simulink model "Main_model"  (R2021b)
settings: Solver=ode23t  StartTime=0.0  StopTime=sim_t_end  RelTol=1e-3
undefined symbols (not defined in the file): ambient_co2, ambient_pressure, ambient_rh, ambient_temp, battery, battery_heat_gen_scale, battery_mass, battery_thermal_mass, cab_air_v_dot, cabin_heater_cmd, cabin_heater_max_power, case_cold_plate_mass, case_cold_plate_thermal_mass, chiller_baffles_n, chiller_tube_length, chiller_tubes_n_rows, compressor_max_m_dot, compressor_ref_m_dot, condenser_air_min_flow_area, condenser_tube_width, const_current, coolant_channel_length, coolant_initial_T, coolant_m_dot, coolant_pipe_cross_sec_area, evaporator_air_cross_sec_area, evaporator_air_min_flow_area, evaporator_tube_width, motor_mc_heat_fraction, n_parallel, power_fraction_rear, ptc_heater_max_power, ptc_heater_thermal_mass, rad_air_v_dot, radiator_air_cross_sec_area, radiator_air_min_flow_area, radiator_tube_width, ref_m_dot, ref_pipe_dia, refrigerant_initial_void_fraction, refrigerant_pipe_cross_sec_area, T_bat_active_cool, T_bat_active_heat, T_bat_passive_cool, T_bat_passive_heat, T_battery_init, T_battery_nom, T_cabin_init, T_cabin_setpoint, T_dcdc_nom, T_DT_high, T_DT_passive_cool, T_DT_whr_active, T_front_gb_nom, T_front_mc_nom, T_front_motor_nom, T_rear_gb_nom, T_rear_mc_nom, T_rear_motor_nom, three_w_valve_max_open_area_factor ... (+3)
libraries: fl_lib x448, nesl_utility x328, SimscapeFluids_lib x134, slpidlib x15, ee_lib x9, simulink x8, LiBatteryElements_lib x4, SignalEditorBlockLib x1
(part 21 of 24)

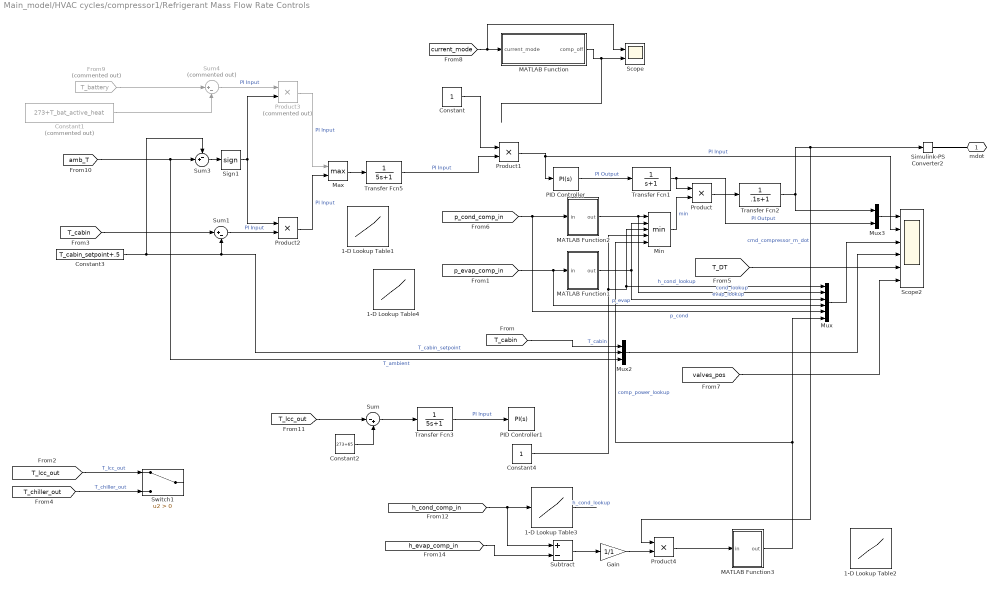
== system Main_model/HVAC cycles/compressor1/Refrigerant Mass Flow Rate Controls  ==
  1-D Lookup Table1 : Lookup_n-D  NumberOfTableDimensions=1  BreakpointsForDimension1=[0,2,2.75,5]  Table=[1,1,0,0]  InternalRulePriority=Speed  RndMeth=Simplest  InputSameDT=on
  1-D Lookup Table2 : Lookup_n-D  NumberOfTableDimensions=1  BreakpointsForDimension1=[0,7.5,8.5,10]  Table=[1,1,0,0]  InternalRulePriority=Speed  RndMeth=Simplest  InputSameDT=on
  1-D Lookup Table3 : Lookup_n-D  NumberOfTableDimensions=1  BreakpointsForDimension1=[400,445,465,500]  Table=[1,1,0,0]  InternalRulePriority=Speed  RndMeth=Simplest  InputSameDT=on
  1-D Lookup Table4 : Lookup_n-D  NumberOfTableDimensions=1  BreakpointsForDimension1=[0,0.08,0.15,1]  Table=[0,0,1,1]  InternalRulePriority=Speed  RndMeth=Simplest  InputSameDT=on
  Constant : Constant
  Constant1 : Constant  Commented=on  Value=273+T_bat_active_heat
  Constant2 : Constant  Value=273+65
  Constant3 : Constant  Value=T_cabin_setpoint+.5
  Constant4 : Constant
  From9 : From  Commented=on  GotoTag=T_battery
  Gain : Gain  Gain=1/1
  MATLAB Function : MATLAB Function  TreatAsAtomicUnit=on
  MATLAB Function1 : MATLAB Function  TreatAsAtomicUnit=on
  MATLAB Function2 : MATLAB Function  TreatAsAtomicUnit=on
  MATLAB Function3 : MATLAB Function  TreatAsAtomicUnit=on
  Max : MinMax  Function=max  Inputs=2
  Min : MinMax  Inputs=5
  Mux : Mux  Inputs=6
  Mux2 : Mux  Inputs=3
  Mux3 : Mux  Inputs=2
  PID Controller : slpidlib/PID Controller  Controller=PI  Form=Parallel  TimeDomain=Continuous-time  UseExternalTs=off  SampleTime=-1  IntegratorMethod=Forward Euler  FilterMethod=Forward Euler  ControllerParametersSource=internal  P=1/7.5*1/5  I=0  D=1  UseFilter=on  N=100  TunerSelectOption=Transfer Function Based (PID Tuner App)  InitialConditionSource=internal  InitialConditionForIntegrator=0  InitialConditionForFilter=0  DifferentiatorICPrevScaledInput=0  ExternalReset=none  TrackingMode=off  Kt=1  LimitOutput=on  SatLimitsSource=internal  UpperSaturationLimit=compressor_max_m_dot  LowerSaturationLimit=0  LinearizeAsGain=on  AntiWindupMode=none  Kb=1  POutMin=[]  POutMax=[]  IOutMin=[]  IOutMax=[]  DOutMin=[]  DOutMax=[]  NOutMin=[]  NOutMax=[]  SumOutMin=[]  SumOutMax=[]  SaturationOutMin=[]  SaturationOutMax=[]  PParamMin=[]  PParamMax=[]  IParamMin=[]  IParamMax=[]  DParamMin=[]  DParamMax=[]  NParamMin=[]  NParamMax=[]  KbParamMin=[]  KbParamMax=[]  KtParamMin=[]  KtParamMax=[]  KbOutMin=[]  KbOutMax=[]  KtOutMin=[]  KtOutMax=[]  IntegratorOutMin=[]  IntegratorOutMax=[]  FilterOutMin=[]  FilterOutMax=[]  SumI1OutMin=[]  SumI1OutMax=[]  SumI2OutMin=[]  SumI2OutMax=[]  SumI3OutMin=[]  SumI3OutMax=[]  SumI4OutMin=[]  SumI4OutMax=[]  SumDOutMin=[]  SumDOutMax=[]  DifferentiatorOutMin=[]  DifferentiatorOutMax=[]  FilterDiffOutCoefMin=[]  FilterDiffOutCoefMax=[]  ReciprocalOutMin=[]  ReciprocalOutMax=[]  SumDenOutMin=[]  SumDenOutMax=[]  SumNumOutMin=[]  SumNumOutMax=[]  DivideOutMin=[]  DivideOutMax=[]  UdiffTsProdOutMin=[]  UdiffTsProdOutMax=[]  NTsProdOutMin=[]  NTsProdOutMax=[]  UintegralTsProdOutMin=[]  UintegralTsProdOutMax=[]  UngainTsProdOutMin=[]  UngainTsProdOutMax=[]  IntegratorContinuousStateAttributes=''  IntegratorStateMustResolveToSignalObject=off  IntegratorRTWStateStorageClass=Auto  FilterContinuousStateAttributes=''  FilterStateMustResolveToSignalObject=off  FilterRTWStateStorageClass=Auto  ParallelPVariant=InternalParameters  IdealPVariant=Disabled  IVariant=InternalParameters  DVariant=Disabled  IntegratorVariant=Continuous  SatVariant=Enabled  AWVariant=Passthrough  PCopyVariant=Disabled  TRVariant=Disabled  FdbkBlocksVariant=Forward  IdealPFdbkVariant=Disabled  SatFdbkVariant=Disabled  DerivativeFilterVariant=Disabled  NVariant=Disabled  NCopyVariant=Disabled_SignalSpec  FilterICVariant=Disabled  IntegratorICVariant=InternalICs  ExternalResetVariant=Disabled  TRSumVariant=Passthrough  SumFdbkVariant=Disabled  SumVariant=Sum_PI  TsampFilterVariant=InternalTs  TsampNgainVariant=Passthrough  TsampIntegralVariant=Passthrough  ExternalSaturationOutDataTypeStr=Inherit: Same as second input
  PID Controller1 : slpidlib/PID Controller  Controller=PI  Form=Ideal  TimeDomain=Continuous-time  UseExternalTs=off  SampleTime=-1  IntegratorMethod=Forward Euler  FilterMethod=Forward Euler  ControllerParametersSource=internal  P=1/20  I=1/5*1/20  D=0  UseFilter=on  N=100  TunerSelectOption=Transfer Function Based (PID Tuner App)  InitialConditionSource=internal  InitialConditionForIntegrator=0  InitialConditionForFilter=0  DifferentiatorICPrevScaledInput=0  ExternalReset=none  TrackingMode=off  Kt=1  LimitOutput=on  SatLimitsSource=internal  UpperSaturationLimit=1  LowerSaturationLimit=0  LinearizeAsGain=on  AntiWindupMode=back-calculation  Kb=1  POutMin=[]  POutMax=[]  IOutMin=[]  IOutMax=[]  DOutMin=[]  DOutMax=[]  NOutMin=[]  NOutMax=[]  SumOutMin=[]  SumOutMax=[]  SaturationOutMin=[]  SaturationOutMax=[]  PParamMin=[]  PParamMax=[]  IParamMin=[]  IParamMax=[]  DParamMin=[]  DParamMax=[]  NParamMin=[]  NParamMax=[]  KbParamMin=[]  KbParamMax=[]  KtParamMin=[]  KtParamMax=[]  KbOutMin=[]  KbOutMax=[]  KtOutMin=[]  KtOutMax=[]  IntegratorOutMin=[]  IntegratorOutMax=[]  FilterOutMin=[]  FilterOutMax=[]  SumI1OutMin=[]  SumI1OutMax=[]  SumI2OutMin=[]  SumI2OutMax=[]  SumI3OutMin=[]  SumI3OutMax=[]  SumI4OutMin=[]  SumI4OutMax=[]  SumDOutMin=[]  SumDOutMax=[]  DifferentiatorOutMin=[]  DifferentiatorOutMax=[]  FilterDiffOutCoefMin=[]  FilterDiffOutCoefMax=[]  ReciprocalOutMin=[]  ReciprocalOutMax=[]  SumDenOutMin=[]  SumDenOutMax=[]  SumNumOutMin=[]  SumNumOutMax=[]  DivideOutMin=[]  DivideOutMax=[]  UdiffTsProdOutMin=[]  UdiffTsProdOutMax=[]  NTsProdOutMin=[]  NTsProdOutMax=[]  UintegralTsProdOutMin=[]  UintegralTsProdOutMax=[]  UngainTsProdOutMin=[]  UngainTsProdOutMax=[]  IntegratorContinuousStateAttributes=''  IntegratorStateMustResolveToSignalObject=off  IntegratorRTWStateStorageClass=Auto  FilterContinuousStateAttributes=''  FilterStateMustResolveToSignalObject=off  FilterRTWStateStorageClass=Auto  ParallelPVariant=Passthrough  IdealPVariant=InternalParameters  IVariant=InternalParameters  DVariant=Disabled  IntegratorVariant=Continuous  SatVariant=Enabled  AWVariant=BackCalculation  PCopyVariant=Disabled  TRVariant=Disabled  FdbkBlocksVariant=Forward  IdealPFdbkVariant=Disabled  SatFdbkVariant=Disabled  DerivativeFilterVariant=Disabled  NVariant=Disabled  NCopyVariant=Disabled_SignalSpec  FilterICVariant=Disabled  IntegratorICVariant=InternalICs  ExternalResetVariant=Disabled  TRSumVariant=Passthrough  SumFdbkVariant=Disabled  SumVariant=Sum_PI  TsampFilterVariant=InternalTs  TsampNgainVariant=Passthrough  TsampIntegralVariant=Passthrough  ExternalSaturationOutDataTypeStr=Inherit: Same as second input
  Product{,1..2,4} (4 alike) : Product
  Product3 : Product  Commented=on
  Scope : Scope  NumInputPorts=2
  Scope2 : Scope  NumInputPorts=6
  Sign1 : Signum
  Simulink-PS Converter2 : nesl_utility/Simulink-PS Converter  PhysicalDomain=network_engine_domain  SubClassName=ps_input  LeftPortType=input  RightPortType=output  PseudoPeriodic=off  Frequencies=[]  NoiseDistribution=none  NoiseParameters=[]  Unit=1  AffineConversion=off  FilteringAndDerivatives=provide  SimscapeFilterOrder=1  InputFilterTimeConstant=0.001  UdotUserProvided=0
      settings: SourceProductBaseCode=PW,SS
  Subtract : Sum  Inputs=+-
  Sum : Sum  Inputs=|-+
  Sum1 : Sum  Inputs=|+-
  Sum3 : Sum  Inputs=-+|
  Sum4 : Sum  Commented=on  Inputs=|+-
  Switch1 : Switch  Criteria=u2 > Threshold
  Transfer Fcn1 : TransferFcn  Denominator=[1 1]
  Transfer Fcn2 : TransferFcn  Denominator=[.1 1]
  Transfer Fcn3 : TransferFcn  Denominator=[5 1]
  Transfer Fcn5 : TransferFcn  Denominator=[5 1]
  mdot : PMIOPort  Side=Right
  wires:
  Transfer Fcn5/1 -> Product1/2  "PI Input"
  [current_mode] -> MATLAB Function/1(current_mode), Scope/1
  Max/1 -> Transfer Fcn5/1
  From9/1 -> Sum4/1
  Constant1/1 -> Sum4/2
  Product3/1 -> Max/1  "PI Input"
  [T_cabin] -> Sum1/1
  Sum1/1 -> Product2/2  "PI Input"
  Sum3/1 -> Sign1/1
  Sign1/1 -> Product2/1, Product3/2
  [T_cabin] -> Mux2/1  "T_cabin"
  [valves_pos] -> Scope2/6
  Mux3/1 -> Scope2/1
  [T_DT] -> Scope2/5
  Mux2/1 -> Scope2/4
  [p_cond_comp_in] -> MATLAB Function2/1(in), Mux/5  "p_cond"
  MATLAB Function2/1(out) -> Mux/2, Min/1  "cond_lookup"
  Constant3/1 -> Mux2/2, Sum1/2, Sum3/1  "T_cabin_setpoint"
  Min/1 -> Product/2  "min"
  [amb_T] -> Sum3/2, Mux2/3  "T_ambient"
  Product1/1 -> Scope2/2, PID Controller/1  "PI Input"
  [T_chiller_out] -> Switch1/3  "T_chiller_out"
  [T_lcc_out] -> Switch1/1  "T_lcc_out"
  MATLAB Function1/1(out) -> Min/2, Mux/3  "evap_lookup"
  Product/1 -> Transfer Fcn2/1
  [p_evap_comp_in] -> MATLAB Function1/1(in), Mux/4  "p_evap"
  PID Controller/1 -> Transfer Fcn1/1  "PI Output"
  Mux/1 -> Scope2/3
  Transfer Fcn1/1 -> Product/1, Mux3/2  "PI Output"
  MATLAB Function/1(comp_off) -> Scope/2
  Constant/1 -> Product1/1
  Transfer Fcn3/1 -> PID Controller1/1  "PI Input"
  [T_lcc_out] -> Sum/1
  Constant2/1 -> Sum/2
  Sum/1 -> Transfer Fcn3/1
  Constant4/1 -> Min/4, Min/3, Mux/1  "h_cond_lookup"
  Sum4/1 -> Product3/1  "PI Input"
  Product2/1 -> Max/2  "PI Input"
  1-D Lookup Table3/1 -> ?  "h_cond_lookup"
  MATLAB Function3/1(out) -> Mux/6, Min/5  "comp_power_lookup"
  Product4/1 -> MATLAB Function3/1(in)
  Gain/1 -> Product4/2
  [h_evap_comp_in] -> Subtract/2
  Subtract/1 -> Gain/1
  [h_cond_comp_in] -> 1-D Lookup Table3/1, Subtract/1
  Transfer Fcn2/1 -> Simulink-PS Converter2/1, Product4/1, Mux3/1  "cmd_compressor_m_dot"
  connections:
  Simulink-PS Converter2/RConn1 -- mdot/RConn1

== system Main_model/HVAC cycles/compressor1/heat loss ==
  Controlled Temperature Source : fl_lib/Thermal/Thermal Sources/Controlled Temperature Source
  Simulink-PS Converter4 : nesl_utility/Simulink-PS Converter  PhysicalDomain=network_engine_domain  SubClassName=ps_input  LeftPortType=input  RightPortType=output  PseudoPeriodic=off  Frequencies=[]  NoiseDistribution=none  NoiseParameters=[]  Unit=K  AffineConversion=off  FilteringAndDerivatives=provide  SimscapeFilterOrder=1  InputFilterTimeConstant=0.001  UdotUserProvided=0
      settings: SourceProductBaseCode=PW,SS
  Thermal Reference : fl_lib/Thermal/Thermal Elements/Thermal Reference
  Thermal Resistor : ee_lib/Passive/Thermal/Thermal Resistor  R=.25 K/W  T_specify=off  T_priority=None  T=0 K  T_nominal_specify=off  T_nominal_unit=K  T_nominal_value=1  Q_specify=off  Q_priority=None  Q=0 W  Q_nominal_specify=off  Q_nominal_unit=W  Q_nominal_value=1
      settings: SourceProductBaseCode=PS  InternalSimscapePortConfiguration="{\"Bottom\":[],\"Left\":[{\"id\":\"A\",\"label\":\"A\",\"type\":\"foundation.thermal.thermal\"}],\"Right\":[{\"id\":\"B\",\"label\":\"B\",\"type\":\"foundation.thermal.thermal\"}],\"Top\":[]}"
  heat loss : fl_lib/Two-Phase Fluid/Elements/Pipe (2P)  length=.2 m  area=refrigerant_pipe_cross_sec_area m^2  Dh=(4*refrigerant_pipe_cross_sec_area/pi)^.5 m  length_add=0.1 m  roughness=15e-6 m  Re_lam=2000  Re_tur=4000  shape_factor=64  Nu_lam=3.66  inertia=simscape.enum.onoff.off  energy_spec=foundation.enum.energy_spec.void_fraction  p_init=refrigerant_initial_P MPa  T_init=refrigerant_initial_T K  x_init=0.5  alpha_init=refrigerant_initial_void_fraction  h_init=1500 kJ/kg  u_init=1500 kJ/kg  mdot_init=0 kg/s  time_constant=0.1 s
      settings: SourceProductBaseCode=SS  InternalSimscapePortConfiguration="{\"Bottom\":[],\"Left\":[{\"id\":\"A\",\"label\":\"A\",\"type\":\"foundation.two_phase_fluid.two_phase_fluid\"},{\"id\":\"H\",\"label\":\"H\",\"type\":\"foundation.thermal.thermal\"}],\"Right\":[{\"id\":\"B\",\"label\":\"B\",\"type\":\"foundation.two_phase_fluid.two_phase_fluid\"}],\"Top\":[]}"
  1 : PMIOPort  Side=Left
  2 : PMIOPort  Port=2  Side=Right
  wires:
  [amb_T] -> Simulink-PS Converter4/1
  connections:
  Simulink-PS Converter4/RConn1 -- Controlled Temperature Source/RConn1
  Thermal Resistor/RConn1 -- Controlled Temperature Source/LConn1
  heat loss/LConn2 -- Thermal Resistor/LConn1
  Thermal Reference/LConn1 -- Controlled Temperature Source/RConn2
  1/RConn1 -- heat loss/LConn1
  heat loss/RConn1 -- 2/RConn1

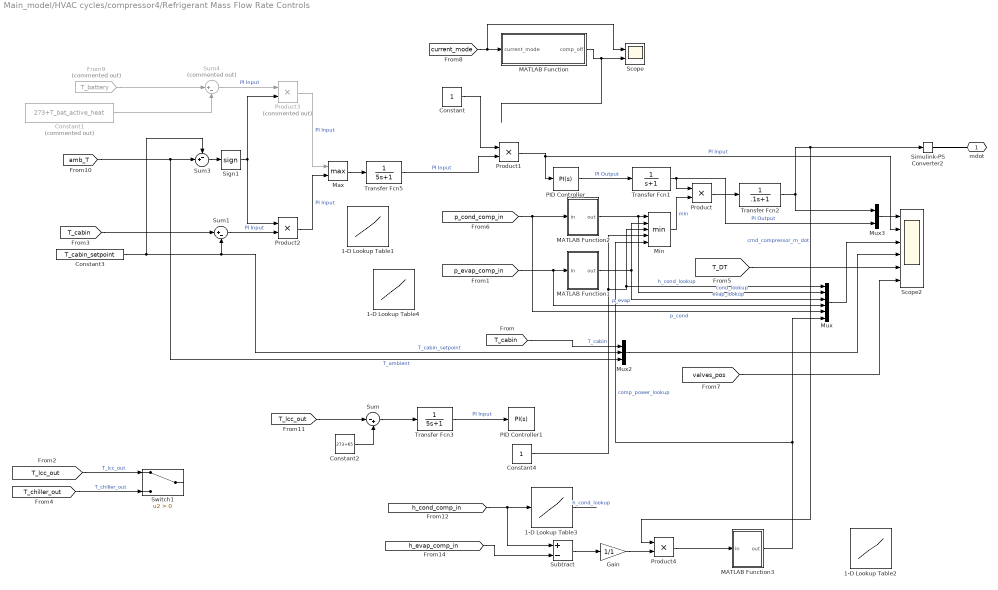
== system Main_model/HVAC cycles/compressor4/Refrigerant Mass Flow Rate Controls  ==
  1-D Lookup Table1 : Lookup_n-D  NumberOfTableDimensions=1  BreakpointsForDimension1=[0,2,2.75,5]  Table=[1,1,0,0]  InternalRulePriority=Speed  RndMeth=Simplest  InputSameDT=on
  1-D Lookup Table2 : Lookup_n-D  NumberOfTableDimensions=1  BreakpointsForDimension1=[0,7.5,8.5,10]  Table=[1,1,0,0]  InternalRulePriority=Speed  RndMeth=Simplest  InputSameDT=on
  1-D Lookup Table3 : Lookup_n-D  NumberOfTableDimensions=1  BreakpointsForDimension1=[400,445,465,500]  Table=[1,1,0,0]  InternalRulePriority=Speed  RndMeth=Simplest  InputSameDT=on
  1-D Lookup Table4 : Lookup_n-D  NumberOfTableDimensions=1  BreakpointsForDimension1=[0,0.08,0.15,1]  Table=[0,0,1,1]  InternalRulePriority=Speed  RndMeth=Simplest  InputSameDT=on
  Constant : Constant
  Constant1 : Constant  Commented=on  Value=273+T_bat_active_heat
  Constant2 : Constant  Value=273+65
  Constant3 : Constant  Value=T_cabin_setpoint
  Constant4 : Constant
  From9 : From  Commented=on  GotoTag=T_battery
  Gain : Gain  Gain=1/1
  MATLAB Function : MATLAB Function  TreatAsAtomicUnit=on
  MATLAB Function1 : MATLAB Function  TreatAsAtomicUnit=on
  MATLAB Function2 : MATLAB Function  TreatAsAtomicUnit=on
  MATLAB Function3 : MATLAB Function  TreatAsAtomicUnit=on
  Max : MinMax  Function=max  Inputs=2
  Min : MinMax  Inputs=5
  Mux : Mux  Inputs=6
  Mux2 : Mux  Inputs=3
  Mux3 : Mux  Inputs=2
  PID Controller : slpidlib/PID Controller  Controller=PI  Form=Parallel  TimeDomain=Continuous-time  UseExternalTs=off  SampleTime=-1  IntegratorMethod=Forward Euler  FilterMethod=Forward Euler  ControllerParametersSource=internal  P=1/2.5*1/5  I=0  D=1  UseFilter=on  N=100  TunerSelectOption=Transfer Function Based (PID Tuner App)  InitialConditionSource=internal  InitialConditionForIntegrator=0  InitialConditionForFilter=0  DifferentiatorICPrevScaledInput=0  ExternalReset=none  TrackingMode=off  Kt=1  LimitOutput=on  SatLimitsSource=internal  UpperSaturationLimit=compressor_max_m_dot  LowerSaturationLimit=0  LinearizeAsGain=on  AntiWindupMode=none  Kb=1  POutMin=[]  POutMax=[]  IOutMin=[]  IOutMax=[]  DOutMin=[]  DOutMax=[]  NOutMin=[]  NOutMax=[]  SumOutMin=[]  SumOutMax=[]  SaturationOutMin=[]  SaturationOutMax=[]  PParamMin=[]  PParamMax=[]  IParamMin=[]  IParamMax=[]  DParamMin=[]  DParamMax=[]  NParamMin=[]  NParamMax=[]  KbParamMin=[]  KbParamMax=[]  KtParamMin=[]  KtParamMax=[]  KbOutMin=[]  KbOutMax=[]  KtOutMin=[]  KtOutMax=[]  IntegratorOutMin=[]  IntegratorOutMax=[]  FilterOutMin=[]  FilterOutMax=[]  SumI1OutMin=[]  SumI1OutMax=[]  SumI2OutMin=[]  SumI2OutMax=[]  SumI3OutMin=[]  SumI3OutMax=[]  SumI4OutMin=[]  SumI4OutMax=[]  SumDOutMin=[]  SumDOutMax=[]  DifferentiatorOutMin=[]  DifferentiatorOutMax=[]  FilterDiffOutCoefMin=[]  FilterDiffOutCoefMax=[]  ReciprocalOutMin=[]  ReciprocalOutMax=[]  SumDenOutMin=[]  SumDenOutMax=[]  SumNumOutMin=[]  SumNumOutMax=[]  DivideOutMin=[]  DivideOutMax=[]  UdiffTsProdOutMin=[]  UdiffTsProdOutMax=[]  NTsProdOutMin=[]  NTsProdOutMax=[]  UintegralTsProdOutMin=[]  UintegralTsProdOutMax=[]  UngainTsProdOutMin=[]  UngainTsProdOutMax=[]  IntegratorContinuousStateAttributes=''  IntegratorStateMustResolveToSignalObject=off  IntegratorRTWStateStorageClass=Auto  FilterContinuousStateAttributes=''  FilterStateMustResolveToSignalObject=off  FilterRTWStateStorageClass=Auto  ParallelPVariant=InternalParameters  IdealPVariant=Disabled  IVariant=InternalParameters  DVariant=Disabled  IntegratorVariant=Continuous  SatVariant=Enabled  AWVariant=Passthrough  PCopyVariant=Disabled  TRVariant=Disabled  FdbkBlocksVariant=Forward  IdealPFdbkVariant=Disabled  SatFdbkVariant=Disabled  DerivativeFilterVariant=Disabled  NVariant=Disabled  NCopyVariant=Disabled_SignalSpec  FilterICVariant=Disabled  IntegratorICVariant=InternalICs  ExternalResetVariant=Disabled  TRSumVariant=Passthrough  SumFdbkVariant=Disabled  SumVariant=Sum_PI  TsampFilterVariant=InternalTs  TsampNgainVariant=Passthrough  TsampIntegralVariant=Passthrough  ExternalSaturationOutDataTypeStr=Inherit: Same as second input
  PID Controller1 : slpidlib/PID Controller  Controller=PI  Form=Ideal  TimeDomain=Continuous-time  UseExternalTs=off  SampleTime=-1  IntegratorMethod=Forward Euler  FilterMethod=Forward Euler  ControllerParametersSource=internal  P=1/20  I=1/5*1/20  D=0  UseFilter=on  N=100  TunerSelectOption=Transfer Function Based (PID Tuner App)  InitialConditionSource=internal  InitialConditionForIntegrator=0  InitialConditionForFilter=0  DifferentiatorICPrevScaledInput=0  ExternalReset=none  TrackingMode=off  Kt=1  LimitOutput=on  SatLimitsSource=internal  UpperSaturationLimit=1  LowerSaturationLimit=0  LinearizeAsGain=on  AntiWindupMode=back-calculation  Kb=1  POutMin=[]  POutMax=[]  IOutMin=[]  IOutMax=[]  DOutMin=[]  DOutMax=[]  NOutMin=[]  NOutMax=[]  SumOutMin=[]  SumOutMax=[]  SaturationOutMin=[]  SaturationOutMax=[]  PParamMin=[]  PParamMax=[]  IParamMin=[]  IParamMax=[]  DParamMin=[]  DParamMax=[]  NParamMin=[]  NParamMax=[]  KbParamMin=[]  KbParamMax=[]  KtParamMin=[]  KtParamMax=[]  KbOutMin=[]  KbOutMax=[]  KtOutMin=[]  KtOutMax=[]  IntegratorOutMin=[]  IntegratorOutMax=[]  FilterOutMin=[]  FilterOutMax=[]  SumI1OutMin=[]  SumI1OutMax=[]  SumI2OutMin=[]  SumI2OutMax=[]  SumI3OutMin=[]  SumI3OutMax=[]  SumI4OutMin=[]  SumI4OutMax=[]  SumDOutMin=[]  SumDOutMax=[]  DifferentiatorOutMin=[]  DifferentiatorOutMax=[]  FilterDiffOutCoefMin=[]  FilterDiffOutCoefMax=[]  ReciprocalOutMin=[]  ReciprocalOutMax=[]  SumDenOutMin=[]  SumDenOutMax=[]  SumNumOutMin=[]  SumNumOutMax=[]  DivideOutMin=[]  DivideOutMax=[]  UdiffTsProdOutMin=[]  UdiffTsProdOutMax=[]  NTsProdOutMin=[]  NTsProdOutMax=[]  UintegralTsProdOutMin=[]  UintegralTsProdOutMax=[]  UngainTsProdOutMin=[]  UngainTsProdOutMax=[]  IntegratorContinuousStateAttributes=''  IntegratorStateMustResolveToSignalObject=off  IntegratorRTWStateStorageClass=Auto  FilterContinuousStateAttributes=''  FilterStateMustResolveToSignalObject=off  FilterRTWStateStorageClass=Auto  ParallelPVariant=Passthrough  IdealPVariant=InternalParameters  IVariant=InternalParameters  DVariant=Disabled  IntegratorVariant=Continuous  SatVariant=Enabled  AWVariant=BackCalculation  PCopyVariant=Disabled  TRVariant=Disabled  FdbkBlocksVariant=Forward  IdealPFdbkVariant=Disabled  SatFdbkVariant=Disabled  DerivativeFilterVariant=Disabled  NVariant=Disabled  NCopyVariant=Disabled_SignalSpec  FilterICVariant=Disabled  IntegratorICVariant=InternalICs  ExternalResetVariant=Disabled  TRSumVariant=Passthrough  SumFdbkVariant=Disabled  SumVariant=Sum_PI  TsampFilterVariant=InternalTs  TsampNgainVariant=Passthrough  TsampIntegralVariant=Passthrough  ExternalSaturationOutDataTypeStr=Inherit: Same as second input
  Product{,1..2,4} (4 alike) : Product
  Product3 : Product  Commented=on
  Scope : Scope  NumInputPorts=2
  Scope2 : Scope  NumInputPorts=6
  Sign1 : Signum
  Simulink-PS Converter2 : nesl_utility/Simulink-PS Converter  PhysicalDomain=network_engine_domain  SubClassName=ps_input  LeftPortType=input  RightPortType=output  PseudoPeriodic=off  Frequencies=[]  NoiseDistribution=none  NoiseParameters=[]  Unit=1  AffineConversion=off  FilteringAndDerivatives=provide  SimscapeFilterOrder=1  InputFilterTimeConstant=0.001  UdotUserProvided=0
      settings: SourceProductBaseCode=PW,SS
  Subtract : Sum  Inputs=+-
  Sum : Sum  Inputs=|-+
  Sum1 : Sum  Inputs=|+-
  Sum3 : Sum  Inputs=-+|
  Sum4 : Sum  Commented=on  Inputs=|+-
  Switch1 : Switch  Criteria=u2 > Threshold
  Transfer Fcn1 : TransferFcn  Denominator=[1 1]
  Transfer Fcn2 : TransferFcn  Denominator=[.1 1]
  Transfer Fcn3 : TransferFcn  Denominator=[5 1]
  Transfer Fcn5 : TransferFcn  Denominator=[5 1]
  mdot : PMIOPort  Side=Right
  wires:
  Transfer Fcn5/1 -> Product1/2  "PI Input"
  [current_mode] -> MATLAB Function/1(current_mode), Scope/1
  Max/1 -> Transfer Fcn5/1
  From9/1 -> Sum4/1
  Constant1/1 -> Sum4/2
  Product3/1 -> Max/1  "PI Input"
  [T_cabin] -> Sum1/1
  Sum1/1 -> Product2/2  "PI Input"
  Sum3/1 -> Sign1/1
  Sign1/1 -> Product2/1, Product3/2
  [T_cabin] -> Mux2/1  "T_cabin"
  [valves_pos] -> Scope2/6
  Mux3/1 -> Scope2/1
  [T_DT] -> Scope2/5
  Mux2/1 -> Scope2/4
  [p_cond_comp_in] -> MATLAB Function2/1(in), Mux/5  "p_cond"
  MATLAB Function2/1(out) -> Mux/2, Min/1  "cond_lookup"
  Constant3/1 -> Mux2/2, Sum1/2, Sum3/1  "T_cabin_setpoint"
  Min/1 -> Product/2  "min"
  [amb_T] -> Sum3/2, Mux2/3  "T_ambient"
  Product1/1 -> Scope2/2, PID Controller/1  "PI Input"
  [T_chiller_out] -> Switch1/3  "T_chiller_out"
  [T_lcc_out] -> Switch1/1  "T_lcc_out"
  MATLAB Function1/1(out) -> Min/2, Mux/3  "evap_lookup"
  Product/1 -> Transfer Fcn2/1
  [p_evap_comp_in] -> MATLAB Function1/1(in), Mux/4  "p_evap"
  PID Controller/1 -> Transfer Fcn1/1  "PI Output"
  Mux/1 -> Scope2/3
  Transfer Fcn1/1 -> Product/1, Mux3/2  "PI Output"
  MATLAB Function/1(comp_off) -> Scope/2
  Constant/1 -> Product1/1
  Transfer Fcn3/1 -> PID Controller1/1  "PI Input"
  [T_lcc_out] -> Sum/1
  Constant2/1 -> Sum/2
  Sum/1 -> Transfer Fcn3/1
  Constant4/1 -> Min/4, Min/3, Mux/1  "h_cond_lookup"
  Sum4/1 -> Product3/1  "PI Input"
  Product2/1 -> Max/2  "PI Input"
  1-D Lookup Table3/1 -> ?  "h_cond_lookup"
  MATLAB Function3/1(out) -> Mux/6, Min/5  "comp_power_lookup"
  Product4/1 -> MATLAB Function3/1(in)
  Gain/1 -> Product4/2
  [h_evap_comp_in] -> Subtract/2
  Subtract/1 -> Gain/1
  [h_cond_comp_in] -> 1-D Lookup Table3/1, Subtract/1
  Transfer Fcn2/1 -> Simulink-PS Converter2/1, Product4/1, Mux3/1  "cmd_compressor_m_dot"
  connections:
  Simulink-PS Converter2/RConn1 -- mdot/RConn1

== system Main_model/HVAC cycles/compressor4/heat loss ==
  Controlled Temperature Source : fl_lib/Thermal/Thermal Sources/Controlled Temperature Source
  Simulink-PS Converter4 : nesl_utility/Simulink-PS Converter  PhysicalDomain=network_engine_domain  SubClassName=ps_input  LeftPortType=input  RightPortType=output  PseudoPeriodic=off  Frequencies=[]  NoiseDistribution=none  NoiseParameters=[]  Unit=K  AffineConversion=off  FilteringAndDerivatives=provide  SimscapeFilterOrder=1  InputFilterTimeConstant=0.001  UdotUserProvided=0
      settings: SourceProductBaseCode=PW,SS
  Thermal Reference : fl_lib/Thermal/Thermal Elements/Thermal Reference
  Thermal Resistor : ee_lib/Passive/Thermal/Thermal Resistor  R=.25 K/W  T_specify=off  T_priority=None  T=0 K  T_nominal_specify=off  T_nominal_unit=K  T_nominal_value=1  Q_specify=off  Q_priority=None  Q=0 W  Q_nominal_specify=off  Q_nominal_unit=W  Q_nominal_value=1
      settings: SourceProductBaseCode=PS  InternalSimscapePortConfiguration="{\"Bottom\":[],\"Left\":[{\"id\":\"A\",\"label\":\"A\",\"type\":\"foundation.thermal.thermal\"}],\"Right\":[{\"id\":\"B\",\"label\":\"B\",\"type\":\"foundation.thermal.thermal\"}],\"Top\":[]}"
  heat loss : fl_lib/Two-Phase Fluid/Elements/Pipe (2P)  length=.2 m  area=refrigerant_pipe_cross_sec_area m^2  Dh=(4*refrigerant_pipe_cross_sec_area/pi)^.5 m  length_add=0.1 m  roughness=15e-6 m  Re_lam=2000  Re_tur=4000  shape_factor=64  Nu_lam=3.66  inertia=simscape.enum.onoff.off  energy_spec=foundation.enum.energy_spec.void_fraction  p_init=refrigerant_initial_P MPa  T_init=refrigerant_initial_T K  x_init=0.5  alpha_init=refrigerant_initial_void_fraction  h_init=1500 kJ/kg  u_init=1500 kJ/kg  mdot_init=0 kg/s  time_constant=0.1 s
      settings: SourceProductBaseCode=SS  InternalSimscapePortConfiguration="{\"Bottom\":[],\"Left\":[{\"id\":\"A\",\"label\":\"A\",\"type\":\"foundation.two_phase_fluid.two_phase_fluid\"},{\"id\":\"H\",\"label\":\"H\",\"type\":\"foundation.thermal.thermal\"}],\"Right\":[{\"id\":\"B\",\"label\":\"B\",\"type\":\"foundation.two_phase_fluid.two_phase_fluid\"}],\"Top\":[]}"
  1 : PMIOPort  Side=Left
  2 : PMIOPort  Port=2  Side=Right
  wires:
  [amb_T] -> Simulink-PS Converter4/1
  connections:
  Simulink-PS Converter4/RConn1 -- Controlled Temperature Source/RConn1
  Thermal Resistor/RConn1 -- Controlled Temperature Source/LConn1
  heat loss/LConn2 -- Thermal Resistor/LConn1
  Thermal Reference/LConn1 -- Controlled Temperature Source/RConn2
  1/RConn1 -- heat loss/LConn1
  heat loss/RConn1 -- 2/RConn1

== system Main_model/HVAC cycles/pump4_1/Coolant Tank1 ==
  Cap (G) : fl_lib/Gas/Elements/Cap (G)  p_specify=off  p_priority=None  p=0.101325 MPa  p_nominal_specify=off  p_nominal_unit=MPa  p_nominal_value=1  T_specify=off  T_priority=None  T=293.15 K  T_nominal_specify=off  T_nominal_unit=K  T_nominal_value=1
      settings: SourceProductBaseCode=SS
  Cap (G)1 : fl_lib/Gas/Elements/Cap (G)  p_specify=off  p_priority=None  p=0.101325 MPa  p_nominal_specify=off  p_nominal_unit=MPa  p_nominal_value=1  T_specify=off  T_priority=None  T=293.15 K  T_nominal_specify=off  T_nominal_unit=K  T_nominal_value=1
      settings: SourceProductBaseCode=SS
  Coolant Tank (G-TL) : SimscapeFluids_lib/Fluid Network Interfaces/Tanks & Accumulators/Tank (G-TL)  volume_total=coolant_tank_vol l  volume_spec=fluids.interfaces.tanks_accumulators.enum.VolumeSpec.Constant  tank_area=coolant_tank_cross_sec_area m^2  level_TLU=[0, 3, 5] m  volume_TLU=[0, 4, 6] m^3  inlet_height=0.1 m  inlet_areas_A1B1=[coolant_pipe_cross_sec_area, coolant_pipe_cross_sec_area] m^2  area_A2=0.01 m^2  g=9.81 m/s^2  p_gas_tank_specify=on  p_gas_tank_priority=High  p_gas_tank=ambient_pressure MPa  p_gas_tank_nominal_specify=off  p_gas_tank_nominal_unit=MPa  p_gas_tank_nominal_value=1  T_gas_tank_specify=on  T_gas_tank_priority=High  T_gas_tank=coolant_initial_T K  T_gas_tank_nominal_specify=off  T_gas_tank_nominal_unit=K  T_gas_tank_nominal_value=1  rho_gas_tank_specify=off  rho_gas_tank_priority=None  rho_gas_tank=1.2 kg/m^3  rho_gas_tank_nominal_specify=off  rho_gas_tank_nominal_unit=kg/m^3  rho_gas_tank_nominal_value=1  T_liquid_tank_specify=on  T_liquid_tank_priority=High  T_liquid_tank=coolant_initial_T K  T_liquid_tank_nominal_specify=off  T_liquid_tank_nominal_unit=K  T_liquid_tank_nominal_value=1  level_specify=on  level_priority=None  level=15 cm  level_nominal_specify=off  level_nominal_unit=m  level_nominal_value=1  volume_liquid_specify=on  volume_liquid_priority=High  volume_liquid=coolant_tank_initial_liq_vol l  volume_liquid_nominal_specify=off  volume_liquid_nominal_unit=m^3  volume_liquid_nominal_value=1  mass_liquid_specify=off  mass_liquid_priority=High  mass_liquid=10 kg  mass_liquid_nominal_specify=off  mass_liquid_nominal_unit=kg  mass_liquid_nominal_value=1  inlet_heights_A2B2=[0, 0] m  inlet_areas_A2B2=[coolant_pipe_cross_sec_area, coolant_pipe_cross_sec_area] m^2  inlet_heights_A2B2C2=[.1, .05, 0] m  inlet_areas_A2B2C2=[.01, .01, .01] m^2
      settings: SourceProductBaseCode=SH  InternalSimscapePortConfiguration="{\"Bottom\":[],\"Left\":[{\"id\":\"A1\",\"label\":\"A1\",\"type\":\"foundation.gas.gas\"},{\"id\":\"B1\",\"label\":\"B1\",\"type\":\"foundation.gas.gas\"},{\"id\":\"A2\",\"label\":\"A2\",\"type\":\"foundation.thermal_liquid.thermal_liquid\"},{\"id\":\"B2\",\"label\":\"B2\",\"type\":\"foundation.thermal_liquid.thermal_liquid\"}],\"Right\":[{\"id\":\"H1\",\"label\":\"H1\",\"type\":\"foundation.thermal.thermal\"},{\"id\":\"H2\",\"label\":\"H2\",\"type\":\"foundation.thermal.thermal\"},{\"id\":\"V_out\",\"label\":\"V\",\"type\":\"output\"},{\"id\":\"L_out\",\"label\":\"L\",\"type\":\"output\"}],\"Top\":[]}"
  PS-Simulink Converter : nesl_utility/PS-Simulink Converter  PhysicalDomain=network_engine_domain  SubClassName=ps_output  LeftPortType=input  RightPortType=output  PseudoPeriodic=off  Frequencies=[]  Unit=inherit  AffineConversion=off
      settings: SourceProductBaseCode=PW,SS
  PS-Simulink Converter1 : nesl_utility/PS-Simulink Converter  PhysicalDomain=network_engine_domain  SubClassName=ps_output  LeftPortType=input  RightPortType=output  PseudoPeriodic=off  Frequencies=[]  Unit=inherit  AffineConversion=off
      settings: SourceProductBaseCode=PW,SS
  Perfect Insulator : fl_lib/Thermal/Thermal Elements/Perfect Insulator  T_specify=off  T_priority=None  T=0 K  T_nominal_specify=off  T_nominal_unit=K  T_nominal_value=1
  "Solver Configuration " : nesl_utility/Solver Configuration  Commented=on  PhysicalDomain=network_engine_domain  SubClassName=solver  LeftPortType=input  RightPortType=generic  Tones=[]  Harmonics=[]  SimulateNoise=off  Profile=off  UseLocalSampling=off  EnableSwitchedLinearOptims=on  FrequencyDomain=off  UseCCode=off  RelTol=0.001  AbsTol=1e-06  MinStep=1e-09  ToWorkspace=off  RevertToSquareIcSolve=off  NumHomotopyIterations=100  PhasorMode=off  PhasorModeNumHarmonics=1  DoDC=off  ResidualTolerance=1e-09  UseLocalSolver=off  LocalSolverChoice=NE_BACKWARD_EULER_ADVANCER  LocalSolverSampleTime=0.001  DoFixedCost=off  MaxNonlinIter=3  MaxModeIter=2  ComputeImpulses=off  ImpulseIterations=2  LinearAlgebra=auto  EquationFormulation=NE_TIME_EF  DelaysMemoryBudget=1024  AutomaticFiltering=on  FilteringTimeConstant=0.001  PartitionStorageMethod=AS_NEEDED  PartitionMemoryBudget=1024  PartitionMethod=ROBUST
      settings: SourceProductBaseCode=PW,SS
  Terminator : Terminator
  Terminator1 : Terminator
  Coolant In : PMIOPort  Side=Left
  Coolant Out : PMIOPort  Port=2  Side=Left
  wires:
  PS-Simulink Converter/1 -> Terminator/1
  PS-Simulink Converter1/1 -> Terminator1/1
  connections:
  Cap (G)1/LConn1 -- Coolant Tank (G-TL)/LConn2
  Perfect Insulator/LConn1 -- Coolant Tank (G-TL)/RConn2 -- Coolant Tank (G-TL)/RConn1
  "Solver Configuration "/RConn1 -- Coolant Tank (G-TL)/LConn4 -- Coolant Out/RConn1
  Coolant Tank (G-TL)/RConn4 -- PS-Simulink Converter1/LConn1
  PS-Simulink Converter/LConn1 -- Coolant Tank (G-TL)/RConn3
  Cap (G)/LConn1 -- Coolant Tank (G-TL)/LConn1
  Coolant In/RConn1 -- Coolant Tank (G-TL)/LConn3

== system Main_model/HVAC cycles/pump4_1/pump ==
  Constant RPM : Constant  Value=1000
  Ideal Angular Velocity Source : fl_lib/Mechanical/Mechanical Sources/Ideal Angular Velocity Source
  Mechanical Rotational Reference : fl_lib/Mechanical/Rotational Elements/Mechanical Rotational Reference
  Simulink-PS Converter : nesl_utility/Simulink-PS Converter  PhysicalDomain=network_engine_domain  SubClassName=ps_input  LeftPortType=input  RightPortType=output  PseudoPeriodic=off  Frequencies=[]  NoiseDistribution=none  NoiseParameters=[]  Unit=rpm  AffineConversion=off  FilteringAndDerivatives=provide  SimscapeFilterOrder=1  InputFilterTimeConstant=0.001  UdotUserProvided=0
      settings: SourceProductBaseCode=PW,SS
  pump : SimscapeFluids_lib/Thermal Liquid/Pumps & Motors/Centrifugal Pump (TL)  pump_parameterization=fluids.thermal_liquid.pumps_motors.enum.CentrifugalPumpParameterization.Nominal  capacity_ref_nominal=pump_nom_capacity lpm  head_ref_nominal=pump_nom_head m  power_ref_nominal=pump_nom_brake_power W  head_ref_max=pump_max_head m  capacity_ref_max=pump_max_capacity lpm  omega_ref_analytic=pump_ref_speed rpm  flow_rate_1D_TLU=[16.67, 30, 40, 53.33, 66.67, 83.33] lpm  head_1D_TLU=[50, 47.5, 45, 40, 35, 25] m  power_1D_TLU=[.6, .75, .85, .93, .98, .99] kW  omega_ref_1D=3500 rpm  rho_ref_1D=998.21 kg/m^3  flow_rate_2D_TLU=[16.67, 23.33, 30, 40, 53.33, 60] lpm  omega_2D_TLU=[2450, 2800, 3150, 3500] rpm  head_2D_TLU=[25, 32.7, 42.5, 50; 24, 31.7, 41, 49; 22.7, 30.5, 39, 47.5; 20, 28, 36, 45; 15.7, 24, 32, 40; 12.5, 21, 29.5, 37.5] m  power_2D_TLU=[.28, .38, .5, .6; .31, .41, .55, .68; .33, .44, .6, .75; .36, .48, .65, .83; .38, .53, .72, .93; .39, .55, .75, .97] kW  rho_ref_2D=998.21 kg/m^3  diameter_ratio=1  mech_orientation=fluids.thermal_liquid.pumps_motors.enum.CentrifugalPumpMechOrientation.Positive  area=coolant_pipe_cross_sec_area m^2
      settings: SourceProductBaseCode=SH  InternalSimscapePortConfiguration="{\"Bottom\":[],\"Left\":[{\"id\":\"A\",\"label\":\"A\",\"type\":\"foundation.thermal_liquid.thermal_liquid\"},{\"id\":\"B\",\"label\":\"B\",\"type\":\"foundation.thermal_liquid.thermal_liquid\"}],\"Right\":[{\"id\":\"R\",\"label\":\"R\",\"type\":\"foundation.mechanical.rotational.rotational\"},{\"id\":\"C\",\"label\":\"C\",\"type\":\"foundation.mechanical.rotational.rotational\"}],\"Top\":[]}"
  Coolant In : PMIOPort  Side=Left
  Coolant Out : PMIOPort  Port=2  Side=Left
  wires:
  Constant RPM/1 -> Simulink-PS Converter/1
  connections:
  Coolant In/RConn1 -- pump/LConn1
  pump/LConn2 -- Coolant Out/RConn1
  Ideal Angular Velocity Source/RConn1 -- Simulink-PS Converter/RConn1
  Ideal Angular Velocity Source/LConn1 -- pump/RConn1
  Mechanical Rotational Reference/LConn1 -- Ideal Angular Velocity Source/RConn2 -- pump/RConn2

== system Main_model/HVAC cycles/pump4_2/Coolant Tank1 ==
  Cap (G) : fl_lib/Gas/Elements/Cap (G)  p_specify=off  p_priority=None  p=0.101325 MPa  p_nominal_specify=off  p_nominal_unit=MPa  p_nominal_value=1  T_specify=off  T_priority=None  T=293.15 K  T_nominal_specify=off  T_nominal_unit=K  T_nominal_value=1
      settings: SourceProductBaseCode=SS
  Cap (G)1 : fl_lib/Gas/Elements/Cap (G)  p_specify=off  p_priority=None  p=0.101325 MPa  p_nominal_specify=off  p_nominal_unit=MPa  p_nominal_value=1  T_specify=off  T_priority=None  T=293.15 K  T_nominal_specify=off  T_nominal_unit=K  T_nominal_value=1
      settings: SourceProductBaseCode=SS
  Coolant Tank (G-TL) : SimscapeFluids_lib/Fluid Network Interfaces/Tanks & Accumulators/Tank (G-TL)  volume_total=coolant_tank_vol l  volume_spec=fluids.interfaces.tanks_accumulators.enum.VolumeSpec.Constant  tank_area=coolant_tank_cross_sec_area m^2  level_TLU=[0, 3, 5] m  volume_TLU=[0, 4, 6] m^3  inlet_height=0.1 m  inlet_areas_A1B1=[coolant_pipe_cross_sec_area, coolant_pipe_cross_sec_area] m^2  area_A2=0.01 m^2  g=9.81 m/s^2  p_gas_tank_specify=on  p_gas_tank_priority=High  p_gas_tank=ambient_pressure MPa  p_gas_tank_nominal_specify=off  p_gas_tank_nominal_unit=MPa  p_gas_tank_nominal_value=1  T_gas_tank_specify=on  T_gas_tank_priority=High  T_gas_tank=coolant_initial_T K  T_gas_tank_nominal_specify=off  T_gas_tank_nominal_unit=K  T_gas_tank_nominal_value=1  rho_gas_tank_specify=off  rho_gas_tank_priority=None  rho_gas_tank=1.2 kg/m^3  rho_gas_tank_nominal_specify=off  rho_gas_tank_nominal_unit=kg/m^3  rho_gas_tank_nominal_value=1  T_liquid_tank_specify=on  T_liquid_tank_priority=High  T_liquid_tank=coolant_initial_T K  T_liquid_tank_nominal_specify=off  T_liquid_tank_nominal_unit=K  T_liquid_tank_nominal_value=1  level_specify=on  level_priority=None  level=15 cm  level_nominal_specify=off  level_nominal_unit=m  level_nominal_value=1  volume_liquid_specify=on  volume_liquid_priority=High  volume_liquid=coolant_tank_initial_liq_vol l  volume_liquid_nominal_specify=off  volume_liquid_nominal_unit=m^3  volume_liquid_nominal_value=1  mass_liquid_specify=off  mass_liquid_priority=High  mass_liquid=10 kg  mass_liquid_nominal_specify=off  mass_liquid_nominal_unit=kg  mass_liquid_nominal_value=1  inlet_heights_A2B2=[0, 0] m  inlet_areas_A2B2=[coolant_pipe_cross_sec_area, coolant_pipe_cross_sec_area] m^2  inlet_heights_A2B2C2=[.1, .05, 0] m  inlet_areas_A2B2C2=[.01, .01, .01] m^2
      settings: SourceProductBaseCode=SH  InternalSimscapePortConfiguration="{\"Bottom\":[],\"Left\":[{\"id\":\"A1\",\"label\":\"A1\",\"type\":\"foundation.gas.gas\"},{\"id\":\"B1\",\"label\":\"B1\",\"type\":\"foundation.gas.gas\"},{\"id\":\"A2\",\"label\":\"A2\",\"type\":\"foundation.thermal_liquid.thermal_liquid\"},{\"id\":\"B2\",\"label\":\"B2\",\"type\":\"foundation.thermal_liquid.thermal_liquid\"}],\"Right\":[{\"id\":\"H1\",\"label\":\"H1\",\"type\":\"foundation.thermal.thermal\"},{\"id\":\"H2\",\"label\":\"H2\",\"type\":\"foundation.thermal.thermal\"},{\"id\":\"V_out\",\"label\":\"V\",\"type\":\"output\"},{\"id\":\"L_out\",\"label\":\"L\",\"type\":\"output\"}],\"Top\":[]}"
  PS-Simulink Converter : nesl_utility/PS-Simulink Converter  PhysicalDomain=network_engine_domain  SubClassName=ps_output  LeftPortType=input  RightPortType=output  PseudoPeriodic=off  Frequencies=[]  Unit=inherit  AffineConversion=off
      settings: SourceProductBaseCode=PW,SS
  PS-Simulink Converter1 : nesl_utility/PS-Simulink Converter  PhysicalDomain=network_engine_domain  SubClassName=ps_output  LeftPortType=input  RightPortType=output  PseudoPeriodic=off  Frequencies=[]  Unit=inherit  AffineConversion=off
      settings: SourceProductBaseCode=PW,SS
  Perfect Insulator : fl_lib/Thermal/Thermal Elements/Perfect Insulator  T_specify=off  T_priority=None  T=0 K  T_nominal_specify=off  T_nominal_unit=K  T_nominal_value=1
  "Solver Configuration " : nesl_utility/Solver Configuration  Commented=on  PhysicalDomain=network_engine_domain  SubClassName=solver  LeftPortType=input  RightPortType=generic  Tones=[]  Harmonics=[]  SimulateNoise=off  Profile=off  UseLocalSampling=off  EnableSwitchedLinearOptims=on  FrequencyDomain=off  UseCCode=off  RelTol=0.001  AbsTol=1e-06  MinStep=1e-09  ToWorkspace=off  RevertToSquareIcSolve=off  NumHomotopyIterations=100  PhasorMode=off  PhasorModeNumHarmonics=1  DoDC=off  ResidualTolerance=1e-09  UseLocalSolver=off  LocalSolverChoice=NE_BACKWARD_EULER_ADVANCER  LocalSolverSampleTime=0.001  DoFixedCost=off  MaxNonlinIter=3  MaxModeIter=2  ComputeImpulses=off  ImpulseIterations=2  LinearAlgebra=auto  EquationFormulation=NE_TIME_EF  DelaysMemoryBudget=1024  AutomaticFiltering=on  FilteringTimeConstant=0.001  PartitionStorageMethod=AS_NEEDED  PartitionMemoryBudget=1024  PartitionMethod=ROBUST
      settings: SourceProductBaseCode=PW,SS
  Terminator : Terminator
  Terminator1 : Terminator
  Coolant In : PMIOPort  Side=Left
  Coolant Out : PMIOPort  Port=2  Side=Left
  wires:
  PS-Simulink Converter/1 -> Terminator/1
  PS-Simulink Converter1/1 -> Terminator1/1
  connections:
  Cap (G)1/LConn1 -- Coolant Tank (G-TL)/LConn2
  Perfect Insulator/LConn1 -- Coolant Tank (G-TL)/RConn2 -- Coolant Tank (G-TL)/RConn1
  "Solver Configuration "/RConn1 -- Coolant Tank (G-TL)/LConn4 -- Coolant Out/RConn1
  Coolant Tank (G-TL)/RConn4 -- PS-Simulink Converter1/LConn1
  PS-Simulink Converter/LConn1 -- Coolant Tank (G-TL)/RConn3
  Cap (G)/LConn1 -- Coolant Tank (G-TL)/LConn1
  Coolant In/RConn1 -- Coolant Tank (G-TL)/LConn3

== system Main_model/HVAC cycles/pump4_2/pump ==
  Constant RPM : Constant  Value=1000
  Ideal Angular Velocity Source : fl_lib/Mechanical/Mechanical Sources/Ideal Angular Velocity Source
  Mechanical Rotational Reference : fl_lib/Mechanical/Rotational Elements/Mechanical Rotational Reference
  Simulink-PS Converter : nesl_utility/Simulink-PS Converter  PhysicalDomain=network_engine_domain  SubClassName=ps_input  LeftPortType=input  RightPortType=output  PseudoPeriodic=off  Frequencies=[]  NoiseDistribution=none  NoiseParameters=[]  Unit=rpm  AffineConversion=off  FilteringAndDerivatives=provide  SimscapeFilterOrder=1  InputFilterTimeConstant=0.001  UdotUserProvided=0
      settings: SourceProductBaseCode=PW,SS
  pump : SimscapeFluids_lib/Thermal Liquid/Pumps & Motors/Centrifugal Pump (TL)  pump_parameterization=fluids.thermal_liquid.pumps_motors.enum.CentrifugalPumpParameterization.Nominal  capacity_ref_nominal=pump_nom_capacity lpm  head_ref_nominal=pump_nom_head m  power_ref_nominal=pump_nom_brake_power W  head_ref_max=pump_max_head m  capacity_ref_max=pump_max_capacity lpm  omega_ref_analytic=pump_ref_speed rpm  flow_rate_1D_TLU=[16.67, 30, 40, 53.33, 66.67, 83.33] lpm  head_1D_TLU=[50, 47.5, 45, 40, 35, 25] m  power_1D_TLU=[.6, .75, .85, .93, .98, .99] kW  omega_ref_1D=3500 rpm  rho_ref_1D=998.21 kg/m^3  flow_rate_2D_TLU=[16.67, 23.33, 30, 40, 53.33, 60] lpm  omega_2D_TLU=[2450, 2800, 3150, 3500] rpm  head_2D_TLU=[25, 32.7, 42.5, 50; 24, 31.7, 41, 49; 22.7, 30.5, 39, 47.5; 20, 28, 36, 45; 15.7, 24, 32, 40; 12.5, 21, 29.5, 37.5] m  power_2D_TLU=[.28, .38, .5, .6; .31, .41, .55, .68; .33, .44, .6, .75; .36, .48, .65, .83; .38, .53, .72, .93; .39, .55, .75, .97] kW  rho_ref_2D=998.21 kg/m^3  diameter_ratio=1  mech_orientation=fluids.thermal_liquid.pumps_motors.enum.CentrifugalPumpMechOrientation.Positive  area=coolant_pipe_cross_sec_area m^2
      settings: SourceProductBaseCode=SH  InternalSimscapePortConfiguration="{\"Bottom\":[],\"Left\":[{\"id\":\"A\",\"label\":\"A\",\"type\":\"foundation.thermal_liquid.thermal_liquid\"},{\"id\":\"B\",\"label\":\"B\",\"type\":\"foundation.thermal_liquid.thermal_liquid\"}],\"Right\":[{\"id\":\"R\",\"label\":\"R\",\"type\":\"foundation.mechanical.rotational.rotational\"},{\"id\":\"C\",\"label\":\"C\",\"type\":\"foundation.mechanical.rotational.rotational\"}],\"Top\":[]}"
  Coolant In : PMIOPort  Side=Left
  Coolant Out : PMIOPort  Port=2  Side=Left
  wires:
  Constant RPM/1 -> Simulink-PS Converter/1
  connections:
  Coolant In/RConn1 -- pump/LConn1
  pump/LConn2 -- Coolant Out/RConn1
  Ideal Angular Velocity Source/RConn1 -- Simulink-PS Converter/RConn1
  Ideal Angular Velocity Source/LConn1 -- pump/RConn1
  Mechanical Rotational Reference/LConn1 -- Ideal Angular Velocity Source/RConn2 -- pump/RConn2

== system Main_model/LCC/Pump/Coolant Tank1 ==
  Cap (G) : fl_lib/Gas/Elements/Cap (G)  p_specify=off  p_priority=None  p=0.101325 MPa  p_nominal_specify=off  p_nominal_unit=MPa  p_nominal_value=1  T_specify=off  T_priority=None  T=293.15 K  T_nominal_specify=off  T_nominal_unit=K  T_nominal_value=1
      settings: SourceProductBaseCode=SS
  Cap (G)1 : fl_lib/Gas/Elements/Cap (G)  p_specify=off  p_priority=None  p=0.101325 MPa  p_nominal_specify=off  p_nominal_unit=MPa  p_nominal_value=1  T_specify=off  T_priority=None  T=293.15 K  T_nominal_specify=off  T_nominal_unit=K  T_nominal_value=1
      settings: SourceProductBaseCode=SS
  Coolant Tank (G-TL) : SimscapeFluids_lib/Fluid Network Interfaces/Tanks & Accumulators/Tank (G-TL)  volume_total=coolant_tank_vol l  volume_spec=fluids.interfaces.tanks_accumulators.enum.VolumeSpec.Constant  tank_area=coolant_tank_cross_sec_area m^2  level_TLU=[0, 3, 5] m  volume_TLU=[0, 4, 6] m^3  inlet_height=0.1 m  inlet_areas_A1B1=[coolant_pipe_cross_sec_area, coolant_pipe_cross_sec_area] m^2  area_A2=0.01 m^2  g=9.81 m/s^2  p_gas_tank_specify=on  p_gas_tank_priority=High  p_gas_tank=ambient_pressure MPa  p_gas_tank_nominal_specify=off  p_gas_tank_nominal_unit=MPa  p_gas_tank_nominal_value=1  T_gas_tank_specify=on  T_gas_tank_priority=High  T_gas_tank=coolant_initial_T K  T_gas_tank_nominal_specify=off  T_gas_tank_nominal_unit=K  T_gas_tank_nominal_value=1  rho_gas_tank_specify=off  rho_gas_tank_priority=None  rho_gas_tank=1.2 kg/m^3  rho_gas_tank_nominal_specify=off  rho_gas_tank_nominal_unit=kg/m^3  rho_gas_tank_nominal_value=1  T_liquid_tank_specify=on  T_liquid_tank_priority=High  T_liquid_tank=coolant_initial_T K  T_liquid_tank_nominal_specify=off  T_liquid_tank_nominal_unit=K  T_liquid_tank_nominal_value=1  level_specify=on  level_priority=None  level=15 cm  level_nominal_specify=off  level_nominal_unit=m  level_nominal_value=1  volume_liquid_specify=on  volume_liquid_priority=High  volume_liquid=coolant_tank_initial_liq_vol l  volume_liquid_nominal_specify=off  volume_liquid_nominal_unit=m^3  volume_liquid_nominal_value=1  mass_liquid_specify=off  mass_liquid_priority=High  mass_liquid=10 kg  mass_liquid_nominal_specify=off  mass_liquid_nominal_unit=kg  mass_liquid_nominal_value=1  inlet_heights_A2B2=[0, 0] m  inlet_areas_A2B2=[coolant_pipe_cross_sec_area, coolant_pipe_cross_sec_area] m^2  inlet_heights_A2B2C2=[.1, .05, 0] m  inlet_areas_A2B2C2=[.01, .01, .01] m^2
      settings: SourceProductBaseCode=SH  InternalSimscapePortConfiguration="{\"Bottom\":[],\"Left\":[{\"id\":\"A1\",\"label\":\"A1\",\"type\":\"foundation.gas.gas\"},{\"id\":\"B1\",\"label\":\"B1\",\"type\":\"foundation.gas.gas\"},{\"id\":\"A2\",\"label\":\"A2\",\"type\":\"foundation.thermal_liquid.thermal_liquid\"},{\"id\":\"B2\",\"label\":\"B2\",\"type\":\"foundation.thermal_liquid.thermal_liquid\"}],\"Right\":[{\"id\":\"H1\",\"label\":\"H1\",\"type\":\"foundation.thermal.thermal\"},{\"id\":\"H2\",\"label\":\"H2\",\"type\":\"foundation.thermal.thermal\"},{\"id\":\"V_out\",\"label\":\"V\",\"type\":\"output\"},{\"id\":\"L_out\",\"label\":\"L\",\"type\":\"output\"}],\"Top\":[]}"
  PS-Simulink Converter : nesl_utility/PS-Simulink Converter  PhysicalDomain=network_engine_domain  SubClassName=ps_output  LeftPortType=input  RightPortType=output  PseudoPeriodic=off  Frequencies=[]  Unit=inherit  AffineConversion=off
      settings: SourceProductBaseCode=PW,SS
  PS-Simulink Converter1 : nesl_utility/PS-Simulink Converter  PhysicalDomain=network_engine_domain  SubClassName=ps_output  LeftPortType=input  RightPortType=output  PseudoPeriodic=off  Frequencies=[]  Unit=inherit  AffineConversion=off
      settings: SourceProductBaseCode=PW,SS
  Perfect Insulator : fl_lib/Thermal/Thermal Elements/Perfect Insulator  T_specify=off  T_priority=None  T=0 K  T_nominal_specify=off  T_nominal_unit=K  T_nominal_value=1
  "Solver Configuration " : nesl_utility/Solver Configuration  Commented=on  PhysicalDomain=network_engine_domain  SubClassName=solver  LeftPortType=input  RightPortType=generic  Tones=[]  Harmonics=[]  SimulateNoise=off  Profile=off  UseLocalSampling=off  EnableSwitchedLinearOptims=on  FrequencyDomain=off  UseCCode=off  RelTol=0.001  AbsTol=1e-06  MinStep=1e-09  ToWorkspace=off  RevertToSquareIcSolve=off  NumHomotopyIterations=100  PhasorMode=off  PhasorModeNumHarmonics=1  DoDC=off  ResidualTolerance=1e-09  UseLocalSolver=off  LocalSolverChoice=NE_BACKWARD_EULER_ADVANCER  LocalSolverSampleTime=0.001  DoFixedCost=off  MaxNonlinIter=3  MaxModeIter=2  ComputeImpulses=off  ImpulseIterations=2  LinearAlgebra=auto  EquationFormulation=NE_TIME_EF  DelaysMemoryBudget=1024  AutomaticFiltering=on  FilteringTimeConstant=0.001  PartitionStorageMethod=AS_NEEDED  PartitionMemoryBudget=1024  PartitionMethod=ROBUST
      settings: SourceProductBaseCode=PW,SS
  Terminator : Terminator
  Terminator1 : Terminator
  Coolant In : PMIOPort  Side=Left
  Coolant Out : PMIOPort  Port=2  Side=Left
  wires:
  PS-Simulink Converter/1 -> Terminator/1
  PS-Simulink Converter1/1 -> Terminator1/1
  connections:
  Cap (G)1/LConn1 -- Coolant Tank (G-TL)/LConn2
  Perfect Insulator/LConn1 -- Coolant Tank (G-TL)/RConn2 -- Coolant Tank (G-TL)/RConn1
  "Solver Configuration "/RConn1 -- Coolant Tank (G-TL)/LConn4 -- Coolant Out/RConn1
  Coolant Tank (G-TL)/RConn4 -- PS-Simulink Converter1/LConn1
  PS-Simulink Converter/LConn1 -- Coolant Tank (G-TL)/RConn3
  Cap (G)/LConn1 -- Coolant Tank (G-TL)/LConn1
  Coolant In/RConn1 -- Coolant Tank (G-TL)/LConn3
